simulink model "PowerSplitHEV_DirectInput"  (R2021a)
settings: Solver=ode23t  StartTime=0.0  StopTime=t_end  RelTol=1e-3  AbsTol=1e-3  EnableMultiTasking=on
PreLoadFcn:
  | PowerSplitHEV_DirectInput_setup
libraries: fl_lib x1, nesl_utility x1
settings Model: FPTRunName=Active  Creator=MathWorks  LastModifiedBy=isaacito
settings SolverCC: AutoScaleAbsTol=off  AlgebraicLoopSolver=TrustRegion
settings DataIOCC: LimitDataPoints=on  MaxDataPoints=15000  SaveFormat=Array  DSMLogging=off  InspectSignalLogs=on
settings OptimizationCC: ExpressionDepthLimit=2147483647  LifeSpan=inf
settings DebuggingCC: UnderspecifiedInitializationDetection=Classic  MergeDetectMultiDrivingBlocksExec=none  StateNameClashWarn=warning  SFUnexpectedBacktrackingDiag=warning  SFNoUnconditionalDefaultTransitionDiag=warning  SFExecutionAtInitializationDiag=none  SFMachineParentedDataDiag=warning  ArithmeticOperatorsInVariantConditions=warning
settings HardwareCC: ProdBitPerPointer=32  ProdBitPerSizeT=32  ProdBitPerPtrDiffT=32  ProdLargestAtomicFloat=None  ProdIntDivRoundTo=Undefined  ProdEndianess=Unspecified  ProdWordSize=32  ProdHWDeviceType=32-bit Generic
settings ModelReferenceCC: PropagateSignalLabelsOutOfModel=off
settings SFSimCC: SimUseLocalCustomCode=off  CustomCodeUndefinedFunction=UseInterfaceOnly
settings RTWCC: RTWUseLocalCustomCode=off
settings CodeAppCC: StateflowObjectComments=on
settings GRTTargetCC: TargetLangStandard=C89/C90 (ANSI)  CombineOutputUpdateFcns=off  GRTInterface=on
settings ConfigComp: CovMetricSettings=dw  CovSaveCumulativeToWorkspaceVar=on  CovSaveSingleToWorkspaceVar=on  CovExternalEMLEnable=off
settings SimscapeCC: SimscapeLogType=all  SimscapeLogSimulationStatistics=on  SimscapeLogName=logoutssc  SimscapeLogLimitData=off  SimscapeLogDataHistory=10000

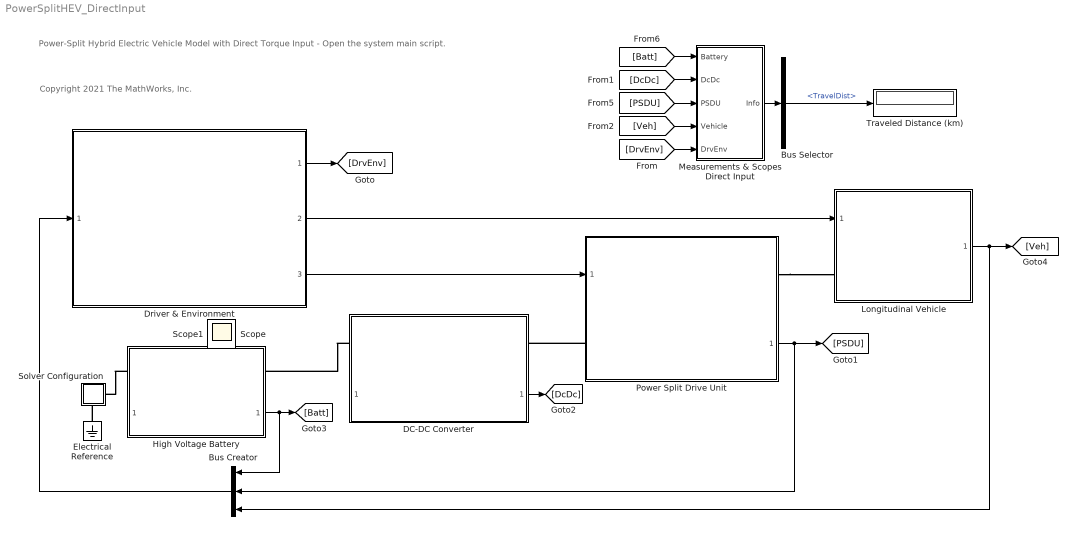
== system PowerSplitHEV_DirectInput ==
  note: Power-Split Hybrid Electric Vehicle Model with Direct Torque Input
      | - Open the system main script.
  note: Copyright 2021 The MathWorks, Inc.
  Bus Creator : BusCreator  Inputs=3
  Bus Selector : BusSelector  OutputSignals=TravelDist
  DC-DC Converter : Subsystem  ReferencedSubsystem=DcDcConverterBasic_refsub
      settings: PortSchema="{\"entries\":[{\"content\":{\"sides\":[{\"content\":{\"connectorIds\":[\"LConn1\",\"In1\"]},\"type\":\"ConnectorPlacement.EquallySpacedRectSide\",\"uuid\":\"9fe8411b-04be-463e-9924-e5b159c802ea\"},{\"content\":{\"connectorIds\":[\"RConn1\",\"Out1\"],\"side\":\"RIGHT\"},\"type\":\"ConnectorPlacement.EquallySpacedRectSide\",\"uuid\":\"f74ab51b-f871-4eba-ad48-2355a260a50e\"},{\"content\":{\"connectorIds\":[],\"side\":\"TOP\"},\"type\":\"ConnectorPlacement.EquallySpacedRectSide\",\"uuid\":\"5fe4b190-e251-4a98-9e87-336539b68eba\"},{\"content\":{\"connectorIds\":[],\"side\":\"HIDDEN\"},\"type\":\"ConnectorPlacement.EquallySpacedRectSide\",\"uuid\":\"70e61028-3020-42d1-b1c6-53691d04cdd7\"}]},\"type\":\"ConnectorPlacement.EquallySpacedConnector\",\"uuid\":\"64b2eeb8-79e5-4be4-98bc-81a0cbd61baa\"}],\"packageUris\":[\"http://schema.mathworks.com/mf0/Connector/R2020b\"],\"version\":\"1.0\"}"
  Driver & Environment : Subsystem  ReferencedSubsystem=PowerSplitHEV_DirectInput_DrvEnv_refsub
  Electrical Reference : fl_lib/Electrical/Electrical Elements/Electrical Reference
  High Voltage Battery : Subsystem  ReferencedSubsystem=BatteryHVBasic_refsub
      settings: PortSchema="{\"entries\":[{\"content\":{\"sides\":[{\"content\":{\"connectorIds\":[\"LConn1\",\"In1\"]},\"type\":\"ConnectorPlacement.EquallySpacedRectSide\",\"uuid\":\"9fe8411b-04be-463e-9924-e5b159c802ea\"},{\"content\":{\"connectorIds\":[\"RConn1\",\"Out1\"],\"side\":\"RIGHT\"},\"type\":\"ConnectorPlacement.EquallySpacedRectSide\",\"uuid\":\"f74ab51b-f871-4eba-ad48-2355a260a50e\"},{\"content\":{\"connectorIds\":[],\"side\":\"TOP\"},\"type\":\"ConnectorPlacement.EquallySpacedRectSide\",\"uuid\":\"5fe4b190-e251-4a98-9e87-336539b68eba\"},{\"content\":{\"connectorIds\":[],\"side\":\"HIDDEN\"},\"type\":\"ConnectorPlacement.EquallySpacedRectSide\",\"uuid\":\"70e61028-3020-42d1-b1c6-53691d04cdd7\"}]},\"type\":\"ConnectorPlacement.EquallySpacedConnector\",\"uuid\":\"64b2eeb8-79e5-4be4-98bc-81a0cbd61baa\"}],\"packageUris\":[\"http://schema.mathworks.com/mf0/Connector/R2020b\"],\"version\":\"1.0\"}"
  Longitudinal Vehicle : Subsystem  ReferencedSubsystem=Vehicle1DBasic_refsub
  Measurements & Scopes Direct Input : Subsystem
  Power Split Drive Unit : Subsystem  ReferencedSubsystem=PowerSplitDriveUnitBasic_refsub
      settings: PortSchema="{\"entries\":[{\"content\":{\"sides\":[{\"content\":{\"connectorIds\":[\"In1\",\"LConn1\"]},\"type\":\"ConnectorPlacement.EquallySpacedRectSide\",\"uuid\":\"974aedaf-bb26-4d59-a293-409346043c39\"},{\"content\":{\"connectorIds\":[\"RConn1\",\"Out1\"],\"side\":\"RIGHT\"},\"type\":\"ConnectorPlacement.EquallySpacedRectSide\",\"uuid\":\"12ed2c12-3442-42d2-9925-d6af8f0a29b3\"},{\"content\":{\"connectorIds\":[],\"side\":\"TOP\"},\"type\":\"ConnectorPlacement.EquallySpacedRectSide\",\"uuid\":\"599325fb-3fa7-4117-9978-1ddfbbeb0247\"},{\"content\":{\"connectorIds\":[],\"side\":\"HIDDEN\"},\"type\":\"ConnectorPlacement.EquallySpacedRectSide\",\"uuid\":\"40453f65-ace7-4c7b-ae3d-0c837e197c38\"}]},\"type\":\"ConnectorPlacement.EquallySpacedConnector\",\"uuid\":\"841da484-ce2c-414e-826b-1cb66c55f7d7\"}],\"packageUris\":[\"http://schema.mathworks.com/mf0/Connector/R2020b\"],\"version\":\"1.0\"}"
  Solver Configuration : Subsystem
      settings: PortSchema="{\"entries\":[{\"content\":{\"sides\":[{\"content\":{\"connectorIds\":[]},\"type\":\"ConnectorPlacement.EquallySpacedRectSide\",\"uuid\":\"4a7e26c2-e9e9-4fea-b605-533b1a682be7\"},{\"content\":{\"connectorIds\":[\"RConn1\"],\"side\":\"RIGHT\"},\"type\":\"ConnectorPlacement.EquallySpacedRectSide\",\"uuid\":\"0210e324-555e-4372-b836-fcc8ab23e933\"},{\"content\":{\"connectorIds\":[],\"side\":\"TOP\"},\"type\":\"ConnectorPlacement.EquallySpacedRectSide\",\"uuid\":\"9bbae011-e6fc-4534-a44f-d79a5697c939\"},{\"content\":{\"connectorIds\":[\"RConn2\"],\"side\":\"BOTTOM\"},\"type\":\"ConnectorPlacement.EquallySpacedRectSide\",\"uuid\":\"d5829c0a-26ea-402d-a1c6-900997ddf1a8\"}]},\"type\":\"ConnectorPlacement.EquallySpacedConnector\",\"uuid\":\"f4e17c65-54c6-42fe-a467-9c6b014b697a\"}],\"packageUris\":[\"http://schema.mathworks.com/mf0/Connector/19700101\"],\"version\":\"1.0\"}"
  Traveled Distance (km) : Display
  Scope : Scope
  Scope1 : Scope
  wires:
  [Batt] -> Measurements & Scopes Direct Input/1(Battery)
  Longitudinal Vehicle/1 -> Bus Creator/3, [Veh]
  [DrvEnv] -> Measurements & Scopes Direct Input/5(DrvEnv)
  Measurements & Scopes Direct Input/1(Info) -> Bus Selector/1
  High Voltage Battery/1 -> Bus Creator/1, [Batt]
  DC-DC Converter/1 -> [DcDc]
  [Veh] -> Measurements & Scopes Direct Input/4(Vehicle)
  [PSDU] -> Measurements & Scopes Direct Input/3(PSDU)
  [DcDc] -> Measurements & Scopes Direct Input/2(DcDc)
  Bus Selector/1 -> Traveled Distance (km)/1  "<TravelDist>"
  Power Split Drive Unit/1 -> Bus Creator/2, [PSDU]
  Driver & Environment/1 -> [DrvEnv]
  Driver & Environment/3 -> Power Split Drive Unit/1
  Driver & Environment/2 -> Longitudinal Vehicle/1
  Bus Creator/1 -> Driver & Environment/1
  connections:
  High Voltage Battery/LConn1 -- Solver Configuration/RConn1
  Electrical Reference/LConn1 -- Solver Configuration/RConn2
  DC-DC Converter/LConn1 -- High Voltage Battery/RConn1
  Power Split Drive Unit/LConn1 -- DC-DC Converter/RConn1
  Power Split Drive Unit/RConn1 -- Longitudinal Vehicle/LConn1

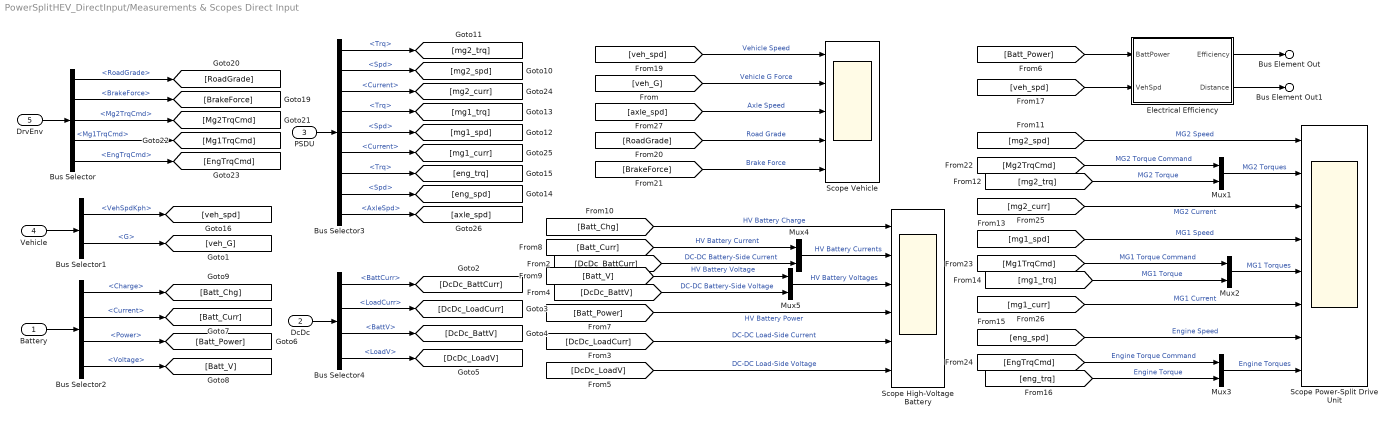
== system PowerSplitHEV_DirectInput/Measurements & Scopes Direct Input ==
  Battery : Inport
  DcDc : Inport  Port=2
  PSDU : Inport  Port=3
  Vehicle : Inport  Port=4
  DrvEnv : Inport  Port=5
  Bus Selector : BusSelector  OutputSignals=RoadGrade,BrakeForce,Mg2TrqCmd,Mg1TrqCmd,EngTrqCmd
  Bus Selector1 : BusSelector  OutputSignals=VehSpdKph,G
  Bus Selector2 : BusSelector  OutputSignals=Charge,Current,Power,Voltage
  Bus Selector3 : BusSelector  OutputSignals=mg2.Trq,mg2.Spd,mg2.Current,mg1.Trq,mg1.Spd,mg1.Current,eng.Trq,eng.Spd,AxleSpd
  Bus Selector4 : BusSelector  OutputSignals=BattCurr,LoadCurr,BattV,LoadV
  Electrical Efficiency : Subsystem
  Mux{1..5} (5 alike) : Mux  Inputs=2
  Scope High-Voltage Battery : Scope  NumInputPorts=6
  Scope Power-Split Drive Unit : Scope  NumInputPorts=8
  Scope Vehicle : Scope  NumInputPorts=5
  Bus Element Out : Outport  PortName=Info  Element=Efficiency
      settings: AttributesFormatString=%<Unit>
  Bus Element Out1 : Outport  PortName=Info  Element=TravelDist
      settings: AttributesFormatString=%<Unit>
  wires:
  [Batt_Power] -> Electrical Efficiency/1(BattPower)
  [veh_spd] -> Electrical Efficiency/2(VehSpd)
  Electrical Efficiency/1(Efficiency) -> Bus Element Out/1
  DrvEnv/1 -> Bus Selector/1
  Vehicle/1 -> Bus Selector1/1
  Bus Selector1/1 -> [veh_spd]  "<VehSpdKph>"
  Bus Selector1/2 -> [veh_G]  "<G>"
  Battery/1 -> Bus Selector2/1
  Bus Selector2/1 -> [Batt_Chg]  "<Charge>"
  Bus Selector2/2 -> [Batt_Curr]  "<Current>"
  Bus Selector2/3 -> [Batt_Power]  "<Power>"
  Bus Selector2/4 -> [Batt_V]  "<Voltage>"
  PSDU/1 -> Bus Selector3/1
  Bus Selector3/1 -> [mg2_trq]  "<Trq>"
  Bus Selector3/2 -> [mg2_spd]  "<Spd>"
  Bus Selector3/3 -> [mg2_curr]  "<Current>"
  Bus Selector3/4 -> [mg1_trq]  "<Trq>"
  Bus Selector3/5 -> [mg1_spd]  "<Spd>"
  Bus Selector3/6 -> [mg1_curr]  "<Current>"
  Bus Selector3/7 -> [eng_trq]  "<Trq>"
  Bus Selector3/8 -> [eng_spd]  "<Spd>"
  DcDc/1 -> Bus Selector4/1
  Bus Selector4/1 -> [DcDc_BattCurr]  "<BattCurr>"
  Bus Selector4/2 -> [DcDc_LoadCurr]  "<LoadCurr>"
  Bus Selector4/3 -> [DcDc_BattV]  "<BattV>"
  Bus Selector4/4 -> [DcDc_LoadV]  "<LoadV>"
  [veh_spd] -> Scope Vehicle/1  "Vehicle Speed"
  [veh_G] -> Scope Vehicle/2  "Vehicle G Force"
  [Mg2TrqCmd] -> Mux1/1  "MG2 Torque Command"
  [mg2_trq] -> Mux1/2  "MG2 Torque"
  [Mg1TrqCmd] -> Mux2/1  "MG1 Torque Command"
  [mg1_trq] -> Mux2/2  "MG1 Torque"
  [EngTrqCmd] -> Mux3/1  "Engine Torque Command"
  [eng_trq] -> Mux3/2  "Engine Torque"
  [Batt_Curr] -> Mux4/1  "HV Battery Current"
  [DcDc_BattCurr] -> Mux4/2  "DC-DC Battery-Side Current"
  [Batt_V] -> Mux5/1  "HV Battery Voltage"
  [DcDc_BattV] -> Mux5/2  "DC-DC Battery-Side Voltage"
  [Batt_Chg] -> Scope High-Voltage Battery/1  "HV Battery Charge"
  Mux4/1 -> Scope High-Voltage Battery/2  "HV Battery Currents"
  Mux5/1 -> Scope High-Voltage Battery/3  "HV Battery Voltages"
  Bus Selector3/9 -> [axle_spd]  "<AxleSpd>"
  [axle_spd] -> Scope Vehicle/3  "Axle Speed"
  Electrical Efficiency/2(Distance) -> Bus Element Out1/1
  Bus Selector/1 -> [RoadGrade]  "<RoadGrade>"
  Bus Selector/2 -> [BrakeForce]  "<BrakeForce>"
  Bus Selector/3 -> [Mg2TrqCmd]  "<Mg2TrqCmd>"
  Bus Selector/4 -> [Mg1TrqCmd]  "<Mg1TrqCmd>"
  Bus Selector/5 -> [EngTrqCmd]  "<EngTrqCmd>"
  [RoadGrade] -> Scope Vehicle/4  "Road Grade"
  [BrakeForce] -> Scope Vehicle/5  "Brake Force"
  [Batt_Power] -> Scope High-Voltage Battery/4  "HV Battery Power"
  [DcDc_LoadCurr] -> Scope High-Voltage Battery/5  "DC-DC Load-Side Current"
  [DcDc_LoadV] -> Scope High-Voltage Battery/6  "DC-DC Load-Side Voltage"
  [mg2_spd] -> Scope Power-Split Drive Unit/1  "MG2 Speed"
  Mux1/1 -> Scope Power-Split Drive Unit/2  "MG2 Torques"
  [mg2_curr] -> Scope Power-Split Drive Unit/3  "MG2 Current"
  [mg1_spd] -> Scope Power-Split Drive Unit/4  "MG1 Speed"
  Mux2/1 -> Scope Power-Split Drive Unit/5  "MG1 Torques"
  [mg1_curr] -> Scope Power-Split Drive Unit/6  "MG1 Current"
  [eng_spd] -> Scope Power-Split Drive Unit/7  "Engine Speed"
  Mux3/1 -> Scope Power-Split Drive Unit/8  "Engine Torques"

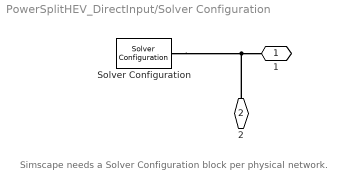
== system PowerSplitHEV_DirectInput/Solver Configuration ==
  note: Simscape needs a Solver Configuration block per physical network.
  Solver Configuration : nesl_utility/Solver Configuration  PhysicalDomain=network_engine_domain  SubClassName=solver  LeftPortType=input  RightPortType=generic  Tones=[]  Harmonics=[]  SimulateNoise=off  Profile=off  UseLocalSampling=off  EnableSwitchedLinearOptims=on  FrequencyDomain=off  UseCCode=off  RelTol=0.001  AbsTol=1e-06  MinStep=1e-09  ToWorkspace=off  RevertToSquareIcSolve=off  NumHomotopyIterations=100  PhasorMode=off  PhasorModeNumHarmonics=1  DoDC=off  ResidualTolerance=1e-9  UseLocalSolver=off  LocalSolverChoice=NE_BACKWARD_EULER_ADVANCER  LocalSolverSampleTime=0.01  DoFixedCost=off  MaxNonlinIter=3  MaxModeIter=2  ComputeImpulses=off  ImpulseIterations=2  LinearAlgebra=auto  EquationFormulation=NE_TIME_EF  DelaysMemoryBudget=1024  AutomaticFiltering=on  FilteringTimeConstant=0.001  PartitionStorageMethod=AS_NEEDED  PartitionMemoryBudget=1024  PartitionMethod=FAST
      settings: AttributesFormatString=Local solver %<UseLocalSolver>  SourceProductBaseCode=PW,SS
  1 : PMIOPort  Side=Right
  2 : PMIOPort  Port=2  Side=Right
  connections:
  Solver Configuration/RConn1 -- 1/RConn1 -- 2/RConn1

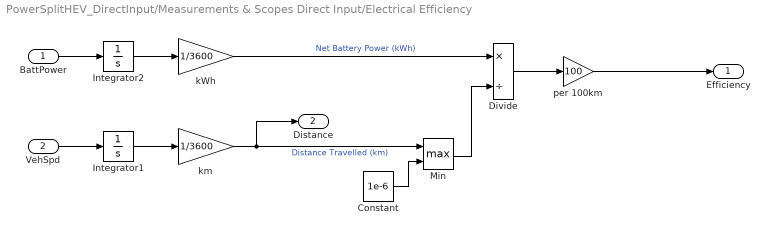
== system PowerSplitHEV_DirectInput/Measurements & Scopes Direct Input/Electrical Efficiency ==
  BattPower : Inport  Unit=kW
      settings: AttributesFormatString=%<Unit>
  VehSpd : Inport  Port=2  Unit=km/hr
      settings: AttributesFormatString=%<Unit>
  Constant : Constant  Value=1e-6
  Divide : Product  Inputs=*/
  Integrator1 : Integrator
      settings: AttributesFormatString=Initial Condition: %<InitialCondition>
  Integrator2 : Integrator
      settings: AttributesFormatString=Initial Condition: %<InitialCondition>
  Min : MinMax  Function=max  Inputs=2
  kWh : Gain  Gain=1/3600
  km : Gain  Gain=1/3600
  per 100km : Gain  Gain=100
  Efficiency : Outport
      settings: AttributesFormatString=%<Unit>
  Distance : Outport  Port=2  Unit=km
  wires:
  per 100km/1 -> Efficiency/1
  Min/1 -> Divide/2
  Integrator1/1 -> km/1
  km/1 -> Min/1, Distance/1  "Distance Travelled (km)"
  Divide/1 -> per 100km/1
  Constant/1 -> Min/2
  kWh/1 -> Divide/1  "Net Battery Power (kWh)"
  Integrator2/1 -> kWh/1
  BattPower/1 -> Integrator2/1
  VehSpd/1 -> Integrator1/1
